simulink model "task1_model"  (R2024a)
settings: Solver=VariableStepAuto  StartTime=0.0  StopTime=10.0  RelTol=1e-3
values from neighbouring files (symbols this model uses):
  P = motor_params()    [build_three_loop_model.m]    (also in task1_openloop.m; task2_speed_step.m; task3_lead_comp.m; task4_position_step.m)
settings Model: Creator=Prima  LastModifiedBy=Prima

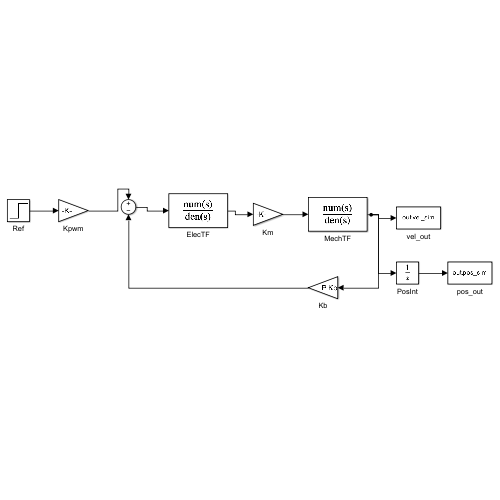
[thumbnail: Simulink's stored preview of the top-level diagram]
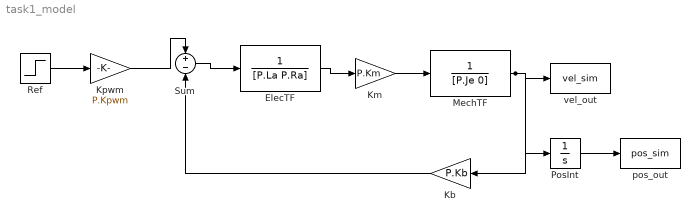
== system task1_model ==
  ElecTF : TransferFcn  Denominator=[P.La P.Ra]
  Kb : Gain  Gain=P.Kb
  Km : Gain  Gain=P.Km
  Kpwm : Gain  Gain=P.Kpwm
  MechTF : TransferFcn  Denominator=[P.Je 0]
  PosInt : Integrator
  Ref : Step  Time=0.05  After=P.Un  SampleTime=0
  Sum : Sum  Inputs=+-
  pos_out : ToWorkspace  VariableName=pos_sim  SaveFormat=Structure With Time  SampleTime=-1
  vel_out : ToWorkspace  VariableName=vel_sim  SaveFormat=Structure With Time  SampleTime=-1
  wires:
  Ref/1 -> Kpwm/1
  Kpwm/1 -> Sum/1
  Sum/1 -> ElecTF/1
  ElecTF/1 -> Km/1
  Km/1 -> MechTF/1
  MechTF/1 -> vel_out/1, PosInt/1, Kb/1
  PosInt/1 -> pos_out/1
  Kb/1 -> Sum/2
